simulink model "demo_simulink_kalman"  (R2018a)
settings: Solver=VariableStepAuto  StartTime=0.0  StopTime=4  RelTol=1e-3
settings Model: Creator=zhaofuhuan  LastModifiedBy=zhaofuhuan

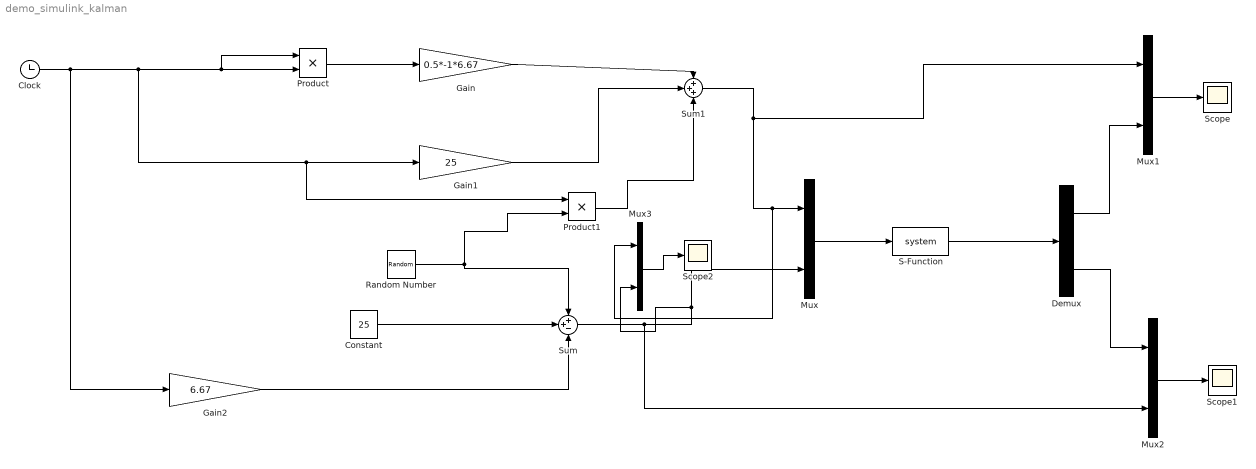
== system demo_simulink_kalman ==
  Clock : Clock
      settings: Decimation=4
  Constant : Constant  Value=25
  Demux : Demux  Outputs=2
  Gain : Gain  Gain=0.5*-1*6.67
  Gain1 : Gain  Gain=25
  Gain2 : Gain  Gain=6.67
  Mux{,1..3} (4 alike) : Mux  Inputs=2
  Product : Product
  Product1 : Product
  Random Number : RandomNumber  Mean=0.5  Variance=0.25  SampleTime=0.1
  S-Function : S-Function  Parameters=6.67  SFunctionDeploymentMode=off  EnableBusSupport=off
  Scope : Scope
  Scope1 : Scope
  Scope2 : Scope
  Sum : Sum  Inputs=++-
  Sum1 : Sum  Inputs=+++
  wires:
  Clock/1 -> Gain2/1, Product1/1, Gain1/1, Product/1, Product/2
  Product/1 -> Gain/1
  Gain/1 -> Sum1/1
  Gain1/1 -> Sum1/2
  Random Number/1 -> Product1/2, Sum/1
  Product1/1 -> Sum1/3
  Gain2/1 -> Sum/3
  Constant/1 -> Sum/2
  Sum1/1 -> Mux1/1, Mux3/1, Mux/1
  Sum/1 -> Mux2/2, Mux3/2, Mux/2
  Mux/1 -> S-Function/1
  S-Function/1 -> Demux/1
  Mux1/1 -> Scope/1
  Demux/1 -> Mux1/2
  Demux/2 -> Mux2/1
  Mux2/1 -> Scope1/1
  Mux3/1 -> Scope2/1
